simulink subsystem "VL53L0"  (R2025b)
settings: Solver=VariableStepAuto  StartTime=0.0  StopTime=10.0  RelTol=1e-3
settings Model: Creator=JesseJabezArendse  LastModifiedBy=JesseJabezArendse

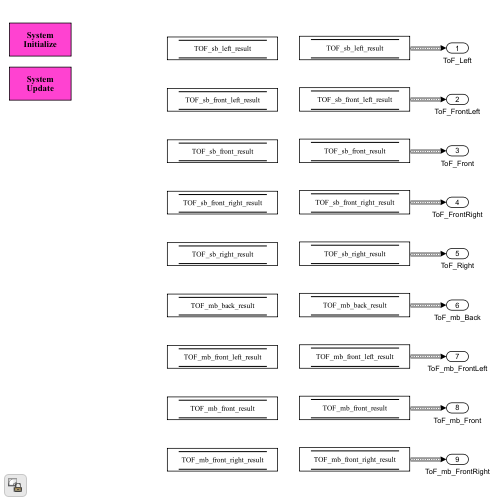
[thumbnail: Simulink's stored preview of the top-level diagram]
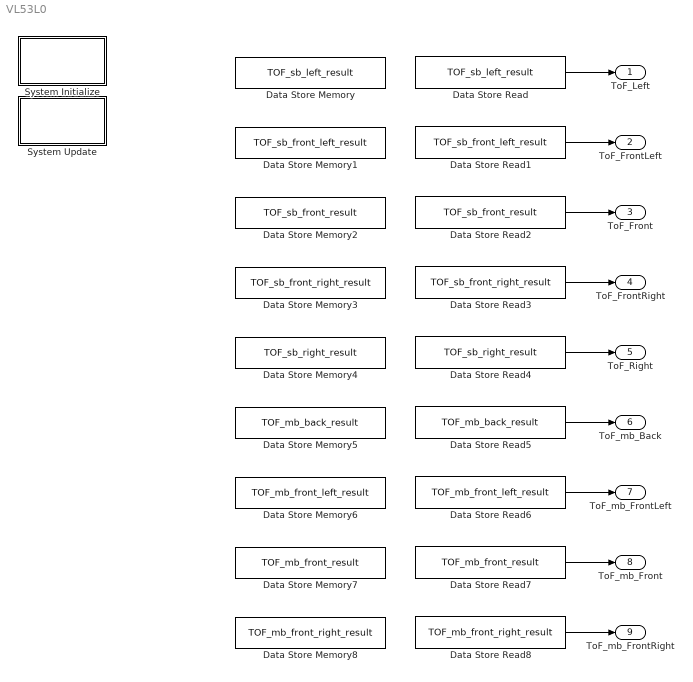
== system VL53L0 ==
  Data Store Memory : DataStoreMemory  DataStoreName=TOF_sb_left_result  WriteAfterWriteMsg=warning  ShowAdditionalParam=off  OutDataTypeStr=Bus: VL53L0_t
  Data Store Memory1 : DataStoreMemory  DataStoreName=TOF_sb_front_left_result  WriteAfterWriteMsg=warning  ShowAdditionalParam=off  OutDataTypeStr=Bus: VL53L0_t
  Data Store Memory2 : DataStoreMemory  DataStoreName=TOF_sb_front_result  WriteAfterWriteMsg=warning  ShowAdditionalParam=off  OutDataTypeStr=Bus: VL53L0_t
  Data Store Memory3 : DataStoreMemory  DataStoreName=TOF_sb_front_right_result  WriteAfterWriteMsg=warning  ShowAdditionalParam=off  OutDataTypeStr=Bus: VL53L0_t
  Data Store Memory4 : DataStoreMemory  DataStoreName=TOF_sb_right_result  WriteAfterWriteMsg=warning  ShowAdditionalParam=off  OutDataTypeStr=Bus: VL53L0_t
  Data Store Memory5 : DataStoreMemory  DataStoreName=TOF_mb_back_result  WriteAfterWriteMsg=warning  ShowAdditionalParam=off  OutDataTypeStr=Bus: VL53L0_t
  Data Store Memory6 : DataStoreMemory  DataStoreName=TOF_mb_front_left_result  WriteAfterWriteMsg=warning  ShowAdditionalParam=off  OutDataTypeStr=Bus: VL53L0_t
  Data Store Memory7 : DataStoreMemory  DataStoreName=TOF_mb_front_result  WriteAfterWriteMsg=warning  ShowAdditionalParam=off  OutDataTypeStr=Bus: VL53L0_t
  Data Store Memory8 : DataStoreMemory  DataStoreName=TOF_mb_front_right_result  WriteAfterWriteMsg=warning  ShowAdditionalParam=off  OutDataTypeStr=Bus: VL53L0_t
  Data Store Read : DataStoreRead  DataStoreName=TOF_sb_left_result  IndexOptions=Index vector (dialog)  Indices=1  OutputSizes=1
  Data Store Read1 : DataStoreRead  DataStoreName=TOF_sb_front_left_result  IndexOptions=Index vector (dialog)  Indices=1  OutputSizes=1
  Data Store Read2 : DataStoreRead  DataStoreName=TOF_sb_front_result  IndexOptions=Index vector (dialog)  Indices=1  OutputSizes=1
  Data Store Read3 : DataStoreRead  DataStoreName=TOF_sb_front_right_result  IndexOptions=Index vector (dialog)  Indices=1  OutputSizes=1
  Data Store Read4 : DataStoreRead  DataStoreName=TOF_sb_right_result  IndexOptions=Index vector (dialog)  Indices=1  OutputSizes=1
  Data Store Read5 : DataStoreRead  DataStoreName=TOF_mb_back_result  IndexOptions=Index vector (dialog)  Indices=1  OutputSizes=1
  Data Store Read6 : DataStoreRead  DataStoreName=TOF_mb_front_left_result  IndexOptions=Index vector (dialog)  Indices=1  OutputSizes=1
  Data Store Read7 : DataStoreRead  DataStoreName=TOF_mb_front_result  IndexOptions=Index vector (dialog)  Indices=1  OutputSizes=1
  Data Store Read8 : DataStoreRead  DataStoreName=TOF_mb_front_right_result  IndexOptions=Index vector (dialog)  Indices=1  OutputSizes=1
  System Initialize : Subsystem  mask(System Initialize){ShowInLibBrowser=0}
      mask prompts: ShowInLibBrowser "Simulink:masks:CustCodeMaskParam1_MP"
      settings: CopyFcn=cccopyfcn(gcb)  OpenFcn=ccopenfcn('System Initialize Function')
      mask Help: eval('feval(''rtwprivate'',''rtwhelpview'',''rtw_sys_initialize_block'')');
      mask Display: disp('System\nInitialize');
  System Update : Subsystem  mask(System Update){ShowInLibBrowser=0}
      mask prompts: ShowInLibBrowser "Simulink:masks:CustCodeMaskParam1_MP"
      settings: CopyFcn=cccopyfcn(gcb)  OpenFcn=ccopenfcn('System Update Function')
      mask Help: eval('feval(''rtwprivate'',''rtwhelpview'',''rtw_sys_update_block'')');
      mask Display: disp('System\nUpdate');
  ToF_Left : Outport
  ToF_FrontLeft : Outport  Port=2
  ToF_Front : Outport  Port=3
  ToF_FrontRight : Outport  Port=4
  ToF_Right : Outport  Port=5
  ToF_mb_Back : Outport  Port=6
  ToF_mb_FrontLeft : Outport  Port=7
  ToF_mb_Front : Outport  Port=8
  ToF_mb_FrontRight : Outport  Port=9
  wires:
  Data Store Read/1 -> ToF_Left/1
  Data Store Read2/1 -> ToF_Front/1
  Data Store Read4/1 -> ToF_Right/1
  Data Store Read1/1 -> ToF_FrontLeft/1
  Data Store Read3/1 -> ToF_FrontRight/1
  Data Store Read5/1 -> ToF_mb_Back/1
  Data Store Read6/1 -> ToF_mb_FrontLeft/1
  Data Store Read7/1 -> ToF_mb_Front/1
  Data Store Read8/1 -> ToF_mb_FrontRight/1

== system VL53L0/System Initialize ==

== system VL53L0/System Update ==
